simulink model "BMS_Out"  (R2022b)
settings: configuration reference "BMS_Sw_CodeGenConfig" (kept outside this file)
undefined symbols (not defined in the file): Ns_Module, NumModules
settings Model: DataDictionary=DD_BMS_Out.sldd  EnableAccessToBaseWorkspace=off  ExtModeTrigDuration=5  Creator=Chirag Patel  LastModifiedBy=Emi
settings ConfigSetRef: SourceName=BMS_Sw_CodeGenConfig

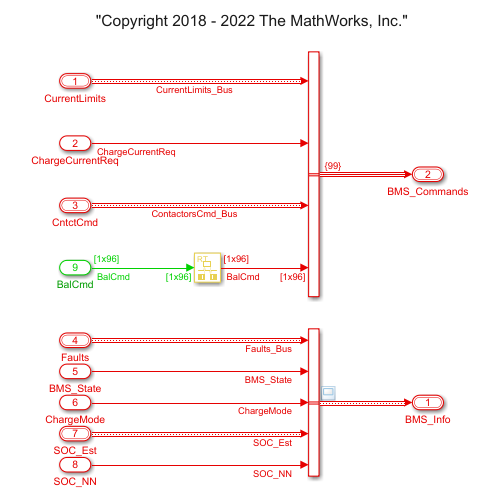
[thumbnail: Simulink's stored preview of the top-level diagram]
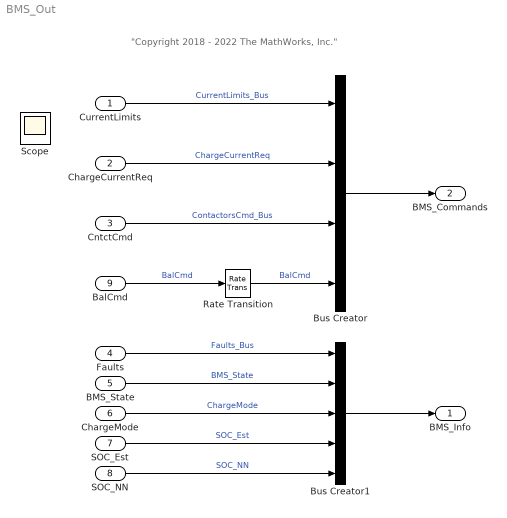
== system BMS_Out ==
  note: "Copyright 2018 - 2022 The MathWorks, Inc."
  CurrentLimits : Inport  OutDataTypeStr=Bus: CurrentLimits  SampleTime=[0.10000000000000001,0]  BusOutputAsStruct=on
  ChargeCurrentReq : Inport  Port=2  OutDataTypeStr=single  PortDimensions=1  SampleTime=[0.10000000000000001,0]
  CntctCmd : Inport  Port=3  OutDataTypeStr=Bus: CntctCmd  SampleTime=[0.10000000000000001,0]  BusOutputAsStruct=on
  Faults : Inport  Port=4  OutDataTypeStr=Bus: Faults  PortDimensions=1  SampleTime=[0.10000000000000001,0]  BusOutputAsStruct=on
  BMS_State : Inport  Port=5  OutDataTypeStr=Enum: BMS_State_Enum  PortDimensions=1  SampleTime=[0.10000000000000001,0]
  ChargeMode : Inport  Port=6
  SOC_Est : Inport  Port=7  OutDataTypeStr=Bus: SOC_Est  SampleTime=[0.10000000000000001,0]  BusOutputAsStruct=on
  SOC_NN : Inport  Port=8
  BalCmd : Inport  Port=9  OutDataTypeStr=boolean  PortDimensions=[1 NumModules*Ns_Module]  SampleTime=[5,0]
  Bus Creator1 : BusCreator  Inputs=5  OutDataTypeStr=Bus: BMS_Info  NonVirtualBus=on
      settings: InheritFromInputs=off
  Bus Creator : BusCreator  Inputs=4  OutDataTypeStr=Bus: BMS_Cmd
  Rate Transition : RateTransition  Integrity=off  Deterministic=off
  BMS_Info : Outport  OutDataTypeStr=Bus: BMS_Info  SampleTime=[0.10000000000000001,0]  BusOutputAsStruct=on
  BMS_Commands : Outport  Port=2  OutDataTypeStr=Bus: BMS_Cmd  SampleTime=[0.10000000000000001,0]  BusOutputAsStruct=on
  Scope : Scope
  wires:
  CntctCmd/1 -> Bus Creator/3  "ContactorsCmd_Bus"
  Faults/1 -> Bus Creator1/1  "Faults_Bus"
  Bus Creator1/1 -> BMS_Info/1
  BalCmd/1 -> Rate Transition/1  "BalCmd"
  Bus Creator/1 -> BMS_Commands/1
  SOC_Est/1 -> Bus Creator1/4  "SOC_Est"
  BMS_State/1 -> Bus Creator1/2  "BMS_State"
  CurrentLimits/1 -> Bus Creator/1  "CurrentLimits_Bus"
  ChargeCurrentReq/1 -> Bus Creator/2  "ChargeCurrentReq"
  Rate Transition/1 -> Bus Creator/4  "BalCmd"
  ChargeMode/1 -> Bus Creator1/3  "ChargeMode"
  SOC_NN/1 -> Bus Creator1/5  "SOC_NN"
